simulink model "inverted_pendulum_2dof"  (R2021b)
settings: Solver=ode45  StartTime=0.0  StopTime=10.0  RelTol=1e-3
settings Model: Creator=lenna  LastModifiedBy=lenna

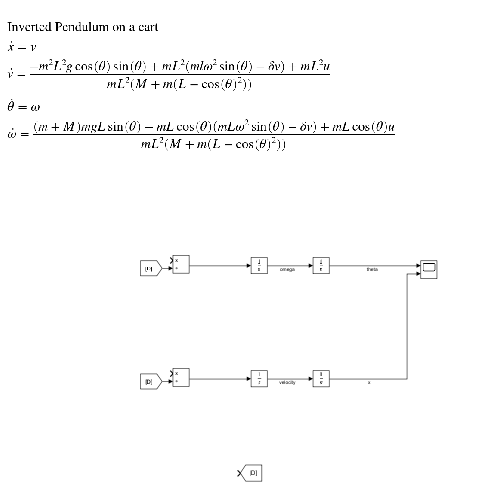
[thumbnail: Simulink's stored preview of the top-level diagram]
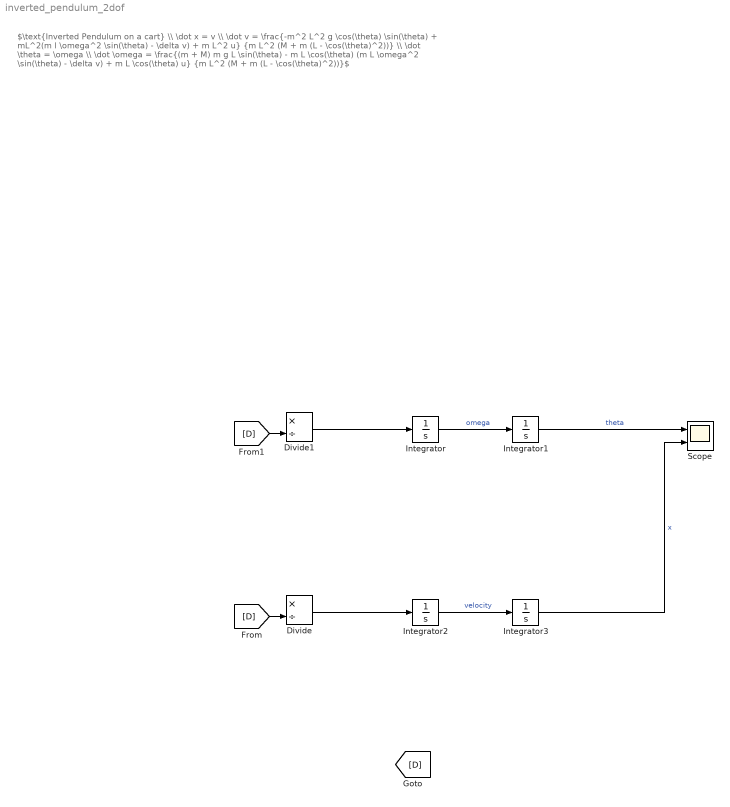
== system inverted_pendulum_2dof ==
  note: $\text{Inverted Pendulum on a cart} \\ \dot x = v \\ \dot v = \frac{-m^2 L^2 g \cos(\theta) \sin(\theta) + mL^2(m l \omega^2 \sin(\theta) - \delta v) + m L^2 u} {m L^2 (M + m (L - \cos(\theta)^2))} \\ \dot \theta = \omega \\ \dot \omega = \frac{(m + M) m g L \sin(\theta) - m L \cos(\theta) (m L \omega^2 \sin(\theta) - \delta v) + m L \cos(\theta) u} {m L^2 (M + m (L - \cos(\theta)^2))}$
  Divide : Product  Inputs=*/
  Divide1 : Product  Inputs=*/
  Integrator{,1..3} (4 alike) : Integrator
  Scope : Scope  NumInputPorts=2
  wires:
  Integrator1/1 -> Scope/1  "theta"
  Integrator/1 -> Integrator1/1  "omega"
  Integrator3/1 -> Scope/2  "x"
  Integrator2/1 -> Integrator3/1  "velocity"
  Divide/1 -> Integrator2/1
  [D] -> Divide/2
  [D] -> Divide1/2
  Divide1/1 -> Integrator/1
